simulink model "sim2"  (R2023a)
settings: Solver=VariableStepAuto  StartTime=0.0  StopTime=50  FixedStep=0.001  RelTol=1e-3
values from neighbouring files (symbols this model uses):
  A = [ 0    1 ... (first row only)    [sim_data2.m]
  B = [0 ... (first row only)    [sim_data2.m]
  C = [1 0]    [sim_data2.m]
  D = [0]    [sim_data2.m]
  dt1 = 1/fs1    (= 0.2)    [sim_data2.m]
  dt2 = 1/fs2    (= 0.0333333333333)    [sim_data2.m]
  dt3 = 1/fs3    (= 0.01)    [sim_data2.m]
  system_disc1 = c2d(system_contin, dt1)    [sim_data2.m]
  system_disc2 = c2d(system_contin, dt2)    [sim_data2.m]
  system_disc3 = c2d(system_contin, dt3)    [sim_data2.m]
settings Model: Creator=ozar  LastModifiedBy=ozar

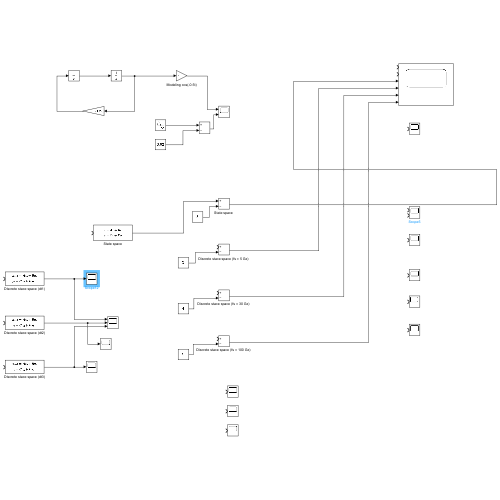
[thumbnail: Simulink's stored preview of the top-level diagram]
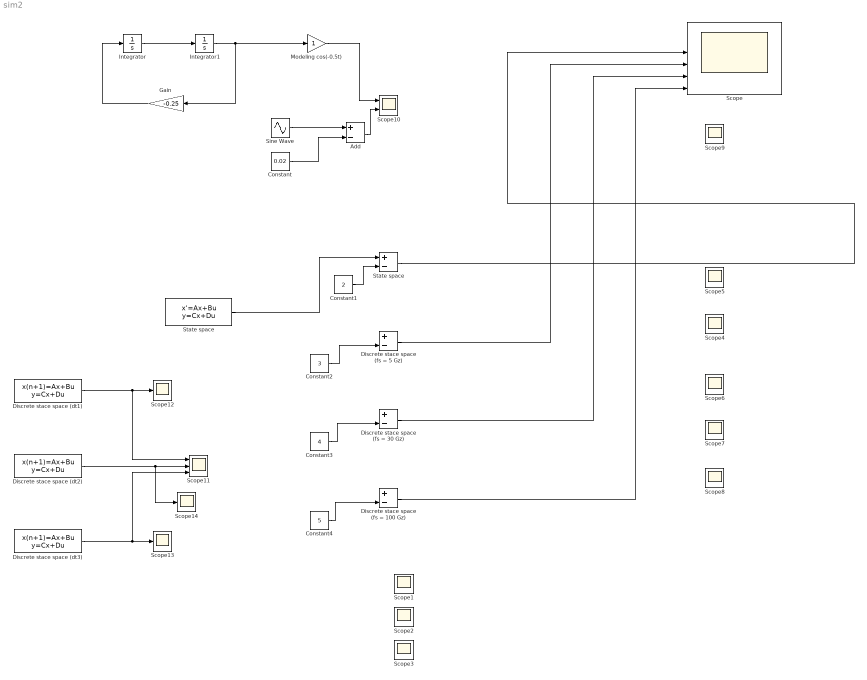
== system sim2 ==
  Add : Sum  Inputs=+-
  Constant : Constant  Value=0.02
  Constant1 : Constant  Value=2
  Constant2 : Constant  Value=3
  Constant3 : Constant  Value=4
  Constant4 : Constant  Value=5
  Discrete stace space (dt1) : DiscreteStateSpace  A=system_disc1.A  B=system_disc1.B  C=system_disc1.C  D=system_disc1.D  InitialCondition=[1; 0]  SampleTime=dt1
  Discrete stace space (dt2) : DiscreteStateSpace  A=system_disc2.A  B=system_disc2.B  C=system_disc2.C  D=system_disc2.D  InitialCondition=[1; 0]  SampleTime=dt2
  Discrete stace space (dt3) : DiscreteStateSpace  A=system_disc3.A  B=system_disc3.B  C=system_disc3.C  D=system_disc3.D  InitialCondition=[1; 0]  SampleTime=dt3
  "Discrete stace space (fs = 100 Gz) " : Sum  Inputs=+-
  "Discrete stace space (fs = 30 Gz) " : Sum  Inputs=+-
  "Discrete stace space (fs = 5 Gz) " : Sum  Inputs=+-
  Gain : Gain  Gain=-0.25
  Integrator : Integrator
  Integrator1 : Integrator  InitialCondition=1
  Modeling cos(-0.5t) : Gain
  Scope : Scope  NumInputPorts=6
  Scope{1..4,6..9,12..14} (11 alike) : Scope
  Scope10 : Scope  NumInputPorts=2
  Scope11 : Scope  NumInputPorts=3
  Scope5 : Scope  NumInputPorts=2
  Sine Wave : Sin  Frequency=0.5  Phase=pi/2  SampleTime=0
  State space : StateSpace  A=A  B=B  C=C  D=D  InitialCondition=[1; 0]
  "State space " : Sum  Inputs=+-
  wires:
  Integrator/1 -> Integrator1/1
  Gain/1 -> Integrator/1
  Integrator1/1 -> Gain/1, Modeling cos(-0.5t)/1
  "State space "/1 -> Scope/3
  State space/1 -> "State space "/1
  Constant1/1 -> "State space "/2
  Constant2/1 -> "Discrete stace space (fs = 5 Gz) "/2
  "Discrete stace space (fs = 5 Gz) "/1 -> Scope/4
  "Discrete stace space (fs = 30 Gz) "/1 -> Scope/5
  Constant3/1 -> "Discrete stace space (fs = 30 Gz) "/2
  Constant4/1 -> "Discrete stace space (fs = 100 Gz) "/2
  "Discrete stace space (fs = 100 Gz) "/1 -> Scope/6
  Modeling cos(-0.5t)/1 -> Scope10/1
  Sine Wave/1 -> Add/1
  Add/1 -> Scope10/2
  Constant/1 -> Add/2
  Discrete stace space (dt2)/1 -> Scope14/1, Scope11/2
  Discrete stace space (dt1)/1 -> Scope12/1, Scope11/1
  Discrete stace space (dt3)/1 -> Scope13/1, Scope11/3
